simulink model "sampleModel2054_2"  (R2023a)
settings: Solver=VariableStepAuto  StartTime=0.0  StopTime=10.0  RelTol=1e-3
libraries: hdlsllib x5, simulink x2
settings Model: Creator=user1  LastModifiedBy=user1

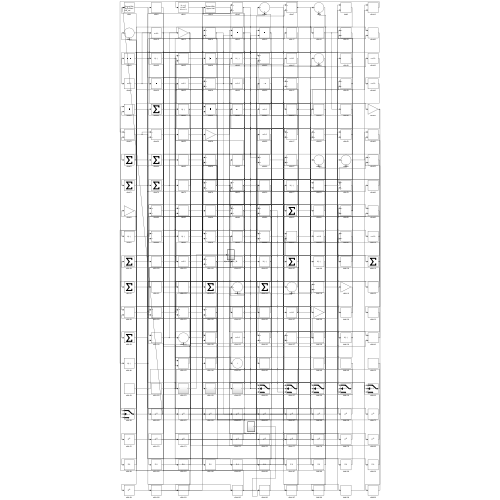
[thumbnail: Simulink's stored preview of the top-level diagram]
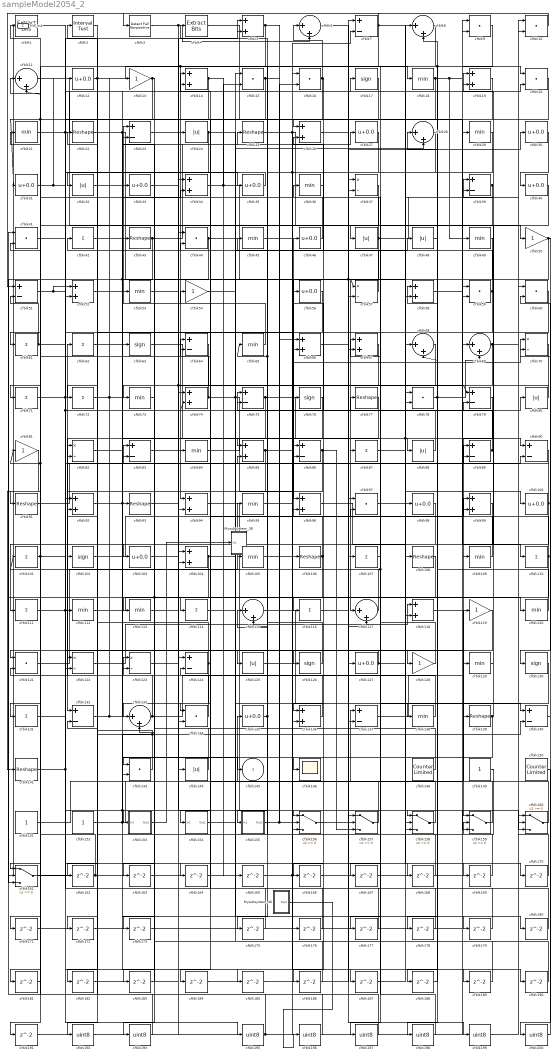
== system sampleModel2054_2 ==
  Mysubsystem_38 : Subsystem  TreatAsAtomicUnit=on  RTWFcnName=Mysubsystem_38
      settings: RTWFcnNameOpts=User specified  RTWFileNameOpts=Use function name
  Mysubsystem_46 : Subsystem  TreatAsAtomicUnit=on  RTWFcnName=Mysubsystem_46
      settings: RTWFcnNameOpts=User specified  RTWFileNameOpts=Use function name
  cfblk1 : simulink/Logic and Bit Operations/Extract Bits  bitsToExtract=Upper half  numBits=8  bitIdxRange=[0 7]  outScalingMode=Preserve fixed-point scaling
      settings: LibrarySourceBlock=|
      | hdlsllib/Logic and Bit
      | Operations/Extract Bits
  cfblk{9..10,15..16,20,41,44,59..60,78,97,121,134,143} (14 alike) : DotProduct  OutDataTypeStr=uint8
  cfblk{12,27,30..31,33,35,40,46,56,98,100,103,127,135} (14 alike) : Bias  Bias=0.0  SaturateOnIntegerOverflow=off
  cfblk{42,61..62,71..72,87,101,107,110..111,114,116,131} (13 alike) : Sum  Inputs=+  OutDataTypeStr=uint8
  cfblk{17,63,76,102,126,130} (6 alike) : Signum
  cfblk{5,14,19,26,34,52,58,66..67,74,85,92,94,96,99,104,118,136} (18 alike) : Sum  OutDataTypeStr=uint8
  cfblk{18,21,29,36,45,49,53,65,73,84,95,105,109,112..113,120,129,138} (18 alike) : MinMax  OutDataTypeStr=uint8
  cfblk{22,25,43,77,91,93,106,108,139,141} (10 alike) : Reshape
  cfblk{6,8,11,28,68..69,115,117,133} (9 alike) : Sum  Inputs=|++  OutDataTypeStr=uint8
  cfblk{13,50,54,81,119,128} (6 alike) : Gain  OutDataTypeStr=uint8
  cfblk{37,57,70,82,122..123} (6 alike) : Product  Inputs=*/  OutDataTypeStr=uint8  RndMeth=Zero  SaturateOnIntegerOverflow=on
  cfblk{7,23,39,51,64,75,79,83,86,89..90,124,132,137,140} (15 alike) : Sum  Inputs=+-  OutDataTypeStr=uint8
  cfblk{24,32,47..48,80,88,125,144} (8 alike) : Abs  OutDataTypeStr=uint8  SaturateOnIntegerOverflow=off
  cfblk146 : Scope
  cfblk148 : hdlsllib/Sources/Counter Limited  uplimit=7  tsamp=-1
  cfblk149 : Constant  OutDataTypeStr=uint8  SampleTime=-1
  cfblk150 : hdlsllib/Sources/Counter Limited  uplimit=7  tsamp=-1
  cfblk151 : Constant  OutDataTypeStr=uint8  SampleTime=-1
  cfblk152 : Constant  OutDataTypeStr=uint8  SampleTime=-1
  cfblk153 : Subsystem
      settings: LibrarySourceBlock=|
      | hdlsllib/Ports &
      | Subsystems/Subsystem
  cfblk154 : Subsystem
      settings: LibrarySourceBlock=|
      | hdlsllib/Ports &
      | Subsystems/Subsystem
  cfblk155 : Subsystem
      settings: LibrarySourceBlock=|
      | hdlsllib/Ports &
      | Subsystems/Subsystem
  cfblk{156..161} (6 alike) : Switch  OutDataTypeStr=uint8  SaturateOnIntegerOverflow=off  InputSameDT=off
  cfblk{162..173,175..191} (29 alike) : Delay  SampleTime=1
  cfblk{192..193,195..200} (8 alike) : DataTypeConversion  OutDataTypeStr=uint8  SaturateOnIntegerOverflow=off  RndMeth=Floor
  cfblk2 : hdlsllib/Logic and Bit Operations/Interval Test  IntervalClosedRight=on  uplimit=0.5  IntervalClosedLeft=on  lowlimit=-0.5  OutDataTypeStr=uint8
  cfblk3 : hdlsllib/Logic and Bit Operations/Detect Fall Nonpositive  vinit=0  OutDataTypeStr=uint8
  cfblk4 : simulink/Logic and Bit Operations/Extract Bits  bitsToExtract=Upper half  numBits=8  bitIdxRange=[0 7]  outScalingMode=Preserve fixed-point scaling
      settings: LibrarySourceBlock=|
      | hdlsllib/Logic and Bit
      | Operations/Extract Bits
  cfblk145 : Outport  OutDataTypeStr=uint8  VectorParamsAs1DForOutWhenUnconnected=off
  Hdl_out : Outport  Port=2  OutDataTypeStr=uint8
  wires:
  cfblk5/1 -> cfblk94/1, cfblk61/1, cfblk66/1
  cfblk127/1 -> cfblk121/1, cfblk80/1
  cfblk79/1 -> cfblk159/1
  cfblk72/1 -> cfblk63/1, cfblk190/1
  cfblk51/1 -> cfblk52/1, cfblk170/1
  cfblk113/1 -> cfblk84/1
  cfblk94/1 -> cfblk156/1
  cfblk70/1 -> cfblk114/1
  cfblk43/1 -> cfblk25/1, cfblk161/2
  cfblk144/1 -> cfblk83/1
  cfblk15/1 -> cfblk31/1, cfblk191/1, cfblk156/2
  cfblk86/1 -> cfblk157/3, cfblk162/1
  cfblk76/1 -> cfblk132/1
  cfblk57/1 -> cfblk42/1
  cfblk110/1 -> cfblk46/1, cfblk122/2
  cfblk41/1 -> cfblk195/1
  cfblk122/1 -> cfblk118/1
  cfblk81/1 -> cfblk141/1
  cfblk62/1 -> cfblk27/1
  cfblk117/1 -> cfblk64/1
  cfblk65/1 -> cfblk23/1
  cfblk44/1 -> cfblk98/1, cfblk57/2, cfblk183/1
  cfblk49/1 -> cfblk96/1
  cfblk59/1 -> cfblk133/1, cfblk36/1
  cfblk16/1 -> cfblk6/1, cfblk146/1, cfblk182/1
  cfblk10/1 -> cfblk51/1
  cfblk3/1 -> cfblk6/2, cfblk117/2
  cfblk30/1 -> cfblk40/1
  cfblk148/1 -> cfblk53/1
  cfblk149/1 -> cfblk159/2
  cfblk13/1 -> cfblk91/1, cfblk133/2
  cfblk20/1 -> cfblk125/1
  cfblk63/1 -> cfblk108/1
  cfblk45/1 -> cfblk47/1
  cfblk112/1 -> cfblk120/1
  cfblk151/1 -> cfblk137/1
  cfblk78/1 -> cfblk69/2, cfblk178/1
  cfblk34/1 -> cfblk117/1, cfblk15/2
  cfblk84/1 -> cfblk90/1
  cfblk83/1 -> cfblk124/1
  cfblk102/1 -> cfblk99/1
  cfblk161/1 -> cfblk16/1, cfblk37/2
  cfblk136/1 -> cfblk62/1
  cfblk32/1 -> cfblk127/1
  cfblk85/1 -> cfblk102/1, cfblk158/3
  cfblk42/1 -> cfblk160/2, cfblk168/1
  cfblk61/1 -> cfblk51/2, cfblk20/2
  cfblk52/1 -> cfblk87/1
  cfblk126/1 -> cfblk4/1
  cfblk159/1 -> cfblk119/1
  cfblk99/1 -> cfblk111/1
  cfblk77/1 -> cfblk113/1
  cfblk25/1 -> cfblk78/1, cfblk140/1
  cfblk95/1 -> cfblk7/2
  cfblk98/1 -> cfblk155/1(In1)
  cfblk128/1 -> cfblk101/1, cfblk33/1
  cfblk106/1 -> cfblk143/1, cfblk44/2
  cfblk26/1 -> cfblk159/3
  cfblk73/1 -> cfblk43/1
  cfblk11/1 -> cfblk78/2
  cfblk111/1 -> cfblk24/1, cfblk153/1(In1)
  cfblk121/1 -> cfblk95/1
  cfblk119/1 -> cfblk131/1
  cfblk8/1 -> cfblk115/2
  cfblk158/1 -> cfblk135/1
  cfblk74/1 -> cfblk106/1, cfblk88/1, cfblk21/1
  cfblk56/1 -> cfblk82/1
  cfblk160/1 -> cfblk58/1
  cfblk18/1 -> cfblk49/1, cfblk20/1, cfblk71/1
  cfblk138/1 -> cfblk75/1
  cfblk64/1 -> cfblk104/2
  cfblk50/1 -> cfblk154/1(In1), cfblk130/1
  cfblk157/1 -> cfblk54/1
  cfblk53/1 -> cfblk79/1, cfblk160/3
  cfblk31/1 -> cfblk12/1, cfblk189/1
  cfblk22/1 -> cfblk57/1, cfblk179/1, cfblk97/1
  cfblk47/1 -> cfblk10/1, cfblk126/1, cfblk26/2
  cfblk124/1 -> cfblk92/2, cfblk163/1
  cfblk75/1 -> cfblk107/1, cfblk134/1
  cfblk134/1 -> cfblk123/1
  cfblk116/1 -> cfblk128/1
  cfblk118/1 -> cfblk29/1
  cfblk104/1 -> cfblk161/3, cfblk193/1, cfblk48/1
  cfblk101/1 -> cfblk85/2, cfblk171/1
  cfblk100/1 -> cfblk86/2, cfblk161/1
  cfblk132/1 -> cfblk34/2, cfblk13/1
  cfblk27/1 -> cfblk137/2
  cfblk33/1 -> cfblk50/1
  cfblk155/1(Out1) -> cfblk70/1, cfblk16/2
  cfblk129/1 -> cfblk89/1
  cfblk21/1 -> cfblk17/1, cfblk26/1, cfblk66/2
  cfblk152/1 -> cfblk59/1, cfblk140/2
  cfblk89/1 -> cfblk75/2, cfblk39/2
  cfblk103/1 -> cfblk76/1
  cfblk88/1 -> cfblk56/1
  cfblk4/1 -> cfblk59/2
  cfblk29/1 -> cfblk96/2, cfblk85/1
  cfblk137/1 -> cfblk9/1
  cfblk69/1 -> cfblk10/2, cfblk116/1
  cfblk54/1 -> cfblk28/2
  cfblk139/1 -> cfblk19/1, cfblk173/1
  cfblk40/1 -> cfblk109/1
  cfblk12/1 -> cfblk72/1, cfblk18/1
  cfblk39/1 -> cfblk19/2, cfblk167/1
  cfblk156/1 -> cfblk30/1
  cfblk93/1 -> cfblk79/2
  cfblk120/1 -> cfblk8/2
  cfblk23/1 -> cfblk74/1
  cfblk35/1 -> cfblk32/1
  cfblk68/1 -> cfblk103/1
  cfblk80/1 -> cfblk73/1
  cfblk1/1 -> cfblk35/1
  cfblk9/1 -> cfblk68/2, cfblk197/1
  cfblk14/1 -> cfblk112/1, cfblk165/1
  cfblk133/1 -> cfblk11/2, cfblk81/1, cfblk118/2
  cfblk46/1 -> cfblk11/1
  cfblk67/1 -> cfblk123/2
  cfblk135/1 -> cfblk105/1, cfblk175/1
  cfblk143/1 -> cfblk22/1, cfblk122/1
  cfblk107/1 -> cfblk67/1
  cfblk71/1 -> cfblk129/1, cfblk74/2, cfblk5/2
  cfblk58/1 -> cfblk110/1
  cfblk109/1 -> cfblk65/1, cfblk45/1
  cfblk154/1(Out1) -> cfblk158/1
  cfblk115/1 -> cfblk138/1
  cfblk140/1 -> cfblk70/2
  cfblk82/1 -> cfblk145/1
  cfblk28/1 -> cfblk136/1
  cfblk96/1 -> cfblk158/2
  cfblk7/1 -> cfblk100/1, cfblk89/2, cfblk134/2, cfblk3/1
  cfblk92/1 -> cfblk93/1, cfblk14/1
  cfblk6/1 -> cfblk37/1
  cfblk141/1 -> cfblk52/2, cfblk185/1
  cfblk97/1 -> cfblk39/1
  cfblk24/1 -> cfblk139/1, cfblk172/1
  cfblk108/1 -> cfblk143/2
  cfblk123/1 -> cfblk5/1
  cfblk91/1 -> cfblk90/2
  cfblk90/1 -> cfblk82/2
  cfblk162/1 -> cfblk1/1, Hdl_out/1
  cfblk163/1 -> cfblk86/1
  cfblk131/1 -> cfblk164/1
  cfblk164/1 -> cfblk157/2
  cfblk165/1 -> cfblk9/2
  cfblk19/1 -> cfblk166/1
  cfblk166/1 -> cfblk68/1
  cfblk167/1 -> cfblk97/2
  cfblk168/1 -> cfblk115/1
  cfblk87/1 -> cfblk169/1
  cfblk169/1 -> cfblk132/2
  cfblk170/1 -> cfblk160/1
  cfblk171/1 -> cfblk58/2
  cfblk172/1 -> cfblk99/2
  cfblk173/1 -> cfblk156/3
  cfblk175/1 -> cfblk64/2
  cfblk105/1 -> cfblk176/1
  cfblk176/1 -> cfblk124/2
  cfblk130/1 -> cfblk177/1
  cfblk177/1 -> cfblk104/1
  cfblk178/1 -> cfblk92/1
  cfblk179/1 -> cfblk14/2
  cfblk114/1 -> cfblk180/1
  cfblk180/1 -> cfblk7/1
  cfblk37/1 -> cfblk181/1
  cfblk181/1 -> cfblk121/2
  cfblk182/1 -> cfblk94/2
  cfblk183/1 -> cfblk23/2
  cfblk17/1 -> cfblk184/1
  cfblk184/1 -> cfblk157/1
  cfblk185/1 -> cfblk67/2
  cfblk36/1 -> cfblk186/1
  cfblk186/1 -> cfblk83/2
  cfblk125/1 -> cfblk187/1
  cfblk187/1 -> cfblk8/1
  cfblk48/1 -> cfblk188/1
  cfblk188/1 -> cfblk28/1
  cfblk189/1 -> cfblk34/1
  cfblk190/1 -> cfblk15/1
  cfblk191/1 -> cfblk136/2
  cfblk2/1 -> cfblk192/1
  cfblk192/1 -> cfblk144/1
  cfblk193/1 -> cfblk2/1
  cfblk195/1 -> cfblk44/1, cfblk69/1
  cfblk196/1 -> cfblk41/1
  cfblk197/1 -> cfblk41/2
  cfblk60/1 -> cfblk198/1
  cfblk198/1 -> cfblk77/1
  cfblk66/1 -> cfblk199/1
  cfblk199/1 -> cfblk60/1
  cfblk150/1 -> cfblk200/1
  cfblk200/1 -> cfblk60/2
  cfblk153/1(Out1) -> Mysubsystem_38/1(In1)
  Mysubsystem_46/1(Out1) -> cfblk196/1

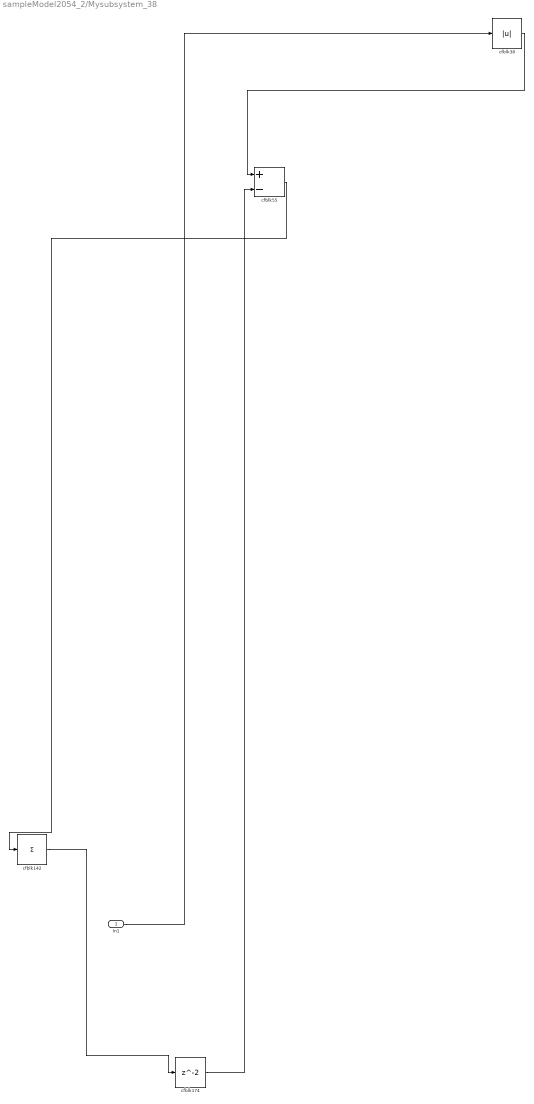
== system sampleModel2054_2/Mysubsystem_38 ==
  In1 : Inport
  cfblk142 : Sum  Inputs=+
  cfblk174 : Delay  SampleTime=1
  cfblk38 : Abs  SaturateOnIntegerOverflow=off
  cfblk55 : Sum  Inputs=+-
  wires:
  cfblk55/1 -> cfblk142/1
  cfblk38/1 -> cfblk55/1
  cfblk142/1 -> cfblk174/1
  cfblk174/1 -> cfblk55/2
  In1/1 -> cfblk38/1

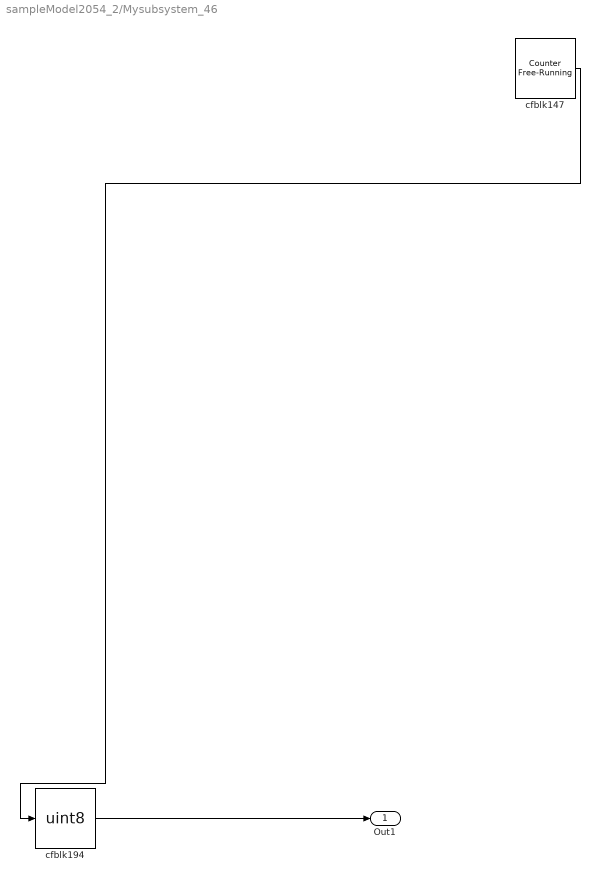
== system sampleModel2054_2/Mysubsystem_46 ==
  cfblk147 : hdlsllib/Sources/Counter Free-Running  NumBits=16  tsamp=-1
  cfblk194 : DataTypeConversion  OutDataTypeStr=uint8  SaturateOnIntegerOverflow=off  RndMeth=Floor
  Out1 : Outport
  wires:
  cfblk147/1 -> cfblk194/1
  cfblk194/1 -> Out1/1

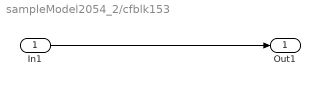
== system sampleModel2054_2/cfblk153 ==
  In1 : Inport
  Out1 : Outport
  wires:
  In1/1 -> Out1/1

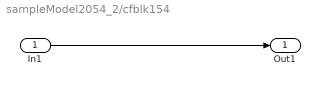
== system sampleModel2054_2/cfblk154 ==
  In1 : Inport
  Out1 : Outport
  wires:
  In1/1 -> Out1/1

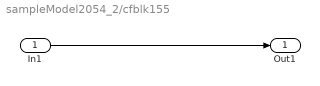
== system sampleModel2054_2/cfblk155 ==
  In1 : Inport
  Out1 : Outport
  wires:
  In1/1 -> Out1/1
